simulink model "gm_sampleModel1931_1_sub"  (R2023a)
settings: Solver=VariableStepAuto  StartTime=0.0  StopTime=10.0  RelTol=1e-3
libraries: simulink x3
settings Model: Creator=user1  LastModifiedBy=user1
settings OptimizationCC: BlockReduction=off  ConditionallyExecuteInputs=off
settings DebuggingCC: InheritedTsInSrcMsg=none

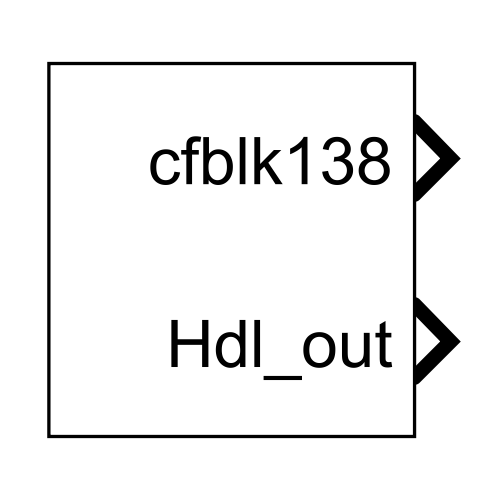
[thumbnail: Simulink's stored preview of the top-level diagram]
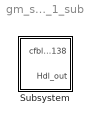
== system gm_sampleModel1931_1_sub ==
  Subsystem : Subsystem

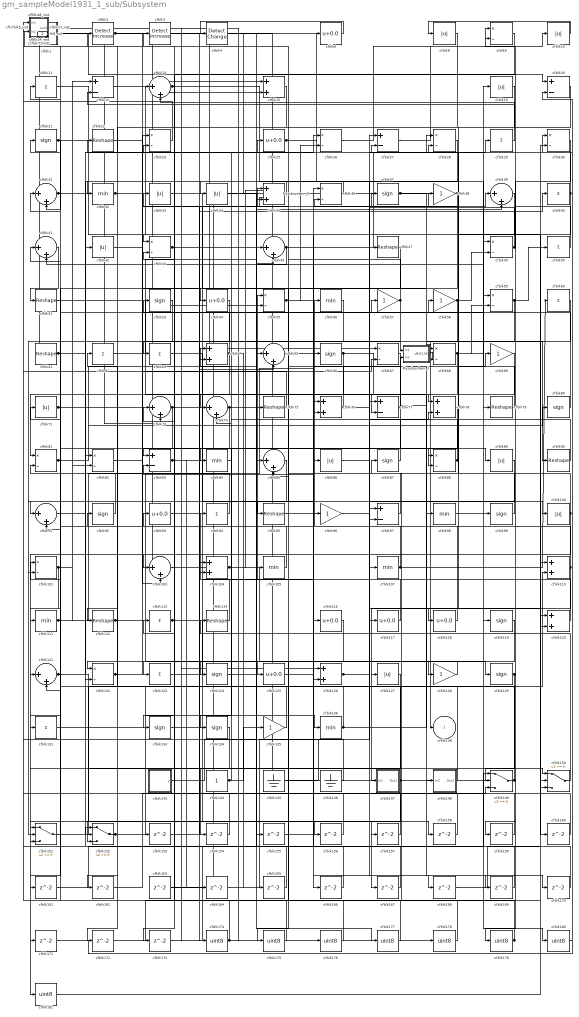
== system gm_sampleModel1931_1_sub/Subsystem ==
  Mysubsystem_1 : Subsystem
  Mysubsystem_5 : Subsystem
  cfblk1 : Subsystem  mask(Compare To Constant){relop=<=, const=double(3), OutDataTypeStr=uint8, ZeroCross=on}
      mask prompts: relop "Simulink:masks:Operator_MP"; const "Simulink:masks:ConstantValue_MP"; OutDataTypeStr "Simulink:masks:OutputDataType_MP"; ZeroCross "Simulink:masks:EnableZerocrossingDetection_MP"
      mask help: Simulink:masks:CompareToConstant_MD
      mask init:
      | OutDataTypeStr = 'uint8';
      | ZeroCross = 'on';
      | blkName = 'sampleModel1931_1_sub/Subsystem/cfblk1';
      | const = double(3);
      | const_str = '3.0';
      | const_val = double(3);
      | relop = '<=';
      | setValue = 'fixdt(0, 8)';
      | str = '<= 3';
      mask TypeOptions relop: == | ~= | < | <= | >= | >
      mask TypeOptions OutDataTypeStr: Simulink:masks:uint8 | Simulink:masks:boolean
      mask Callback ZeroCross: sl('zeroCrossEnable', gcbh);
      mask Display: disp(str)
  cfblk{8,10,19,33..34,42,71,86,89,100,127} (11 alike) : Abs  OutDataTypeStr=uint8  SaturateOnIntegerOverflow=off
  cfblk{9,23,26,28,30,36,43,49,55,59,67..68,81..82,88,101,122} (17 alike) : Product  Inputs=*/  OutDataTypeStr=uint8  RndMeth=Zero  SaturateOnIntegerOverflow=on
  cfblk102_inst : Subsystem
  cfblk{13,31,39,41,45,65,73..74,85,91,103,121} (12 alike) : Sum  Inputs=|++  OutDataTypeStr=uint8
  cfblk{15,35,64,76,78,104,110,120,126} (9 alike) : Sum  OutDataTypeStr=uint8
  cfblk{32,56,84,98,105,107,111,136} (8 alike) : MinMax  OutDataTypeStr=uint8
  cfblk106_inst : Subsystem
  cfblk{11,29,40,50,60,62..63,94,113,123,131} (11 alike) : Sum  Inputs=+  OutDataTypeStr=uint8
  cfblk{22,47,51,61,75,79,90,95,112,114} (10 alike) : Reshape
  cfblk115_inst : Subsystem
  cfblk{6,25,54,93,116..118,125} (8 alike) : Bias  Bias=0.0  SaturateOnIntegerOverflow=off
  cfblk{21,37,53,66,80,87,92,99,119,124,129,133..134} (13 alike) : Signum
  cfblk{12,20,27,77,83,97} (6 alike) : Sum  Inputs=+-  OutDataTypeStr=uint8
  cfblk{38,57..58,69,96,128,135} (7 alike) : Gain  OutDataTypeStr=uint8
  cfblk143 : Subsystem  mask(Counter Free-Running){NumBits=double(16), tsamp=double(-1)}
      mask prompts: NumBits "Simulink:masks:NumberOfBits_MP"; tsamp "Simulink:masks:SampleTime_MP"
      mask help: Simulink:masks:CounterFreeRunning_MD
  cfblk144 : Constant  OutDataTypeStr=uint8  SampleTime=-1
  cfblk145 : Ground
  cfblk146 : Ground
  cfblk147 : Subsystem
  cfblk148 : Subsystem
  cfblk{149..152} (4 alike) : Switch  OutDataTypeStr=uint8  SaturateOnIntegerOverflow=off  InputSameDT=off
  cfblk14_inst : Subsystem
  cfblk{153..173} (21 alike) : Delay  SampleTime=1
  cfblk{174..181} (8 alike) : DataTypeConversion  OutDataTypeStr=uint8  SaturateOnIntegerOverflow=off  RndMeth=Floor
  cfblk17_inst : Subsystem
  cfblk2 : simulink/Logic and Bit Operations/Detect Increase  vinit=0.0  OutDataTypeStr=uint8
      settings: LibrarySourceBlock=|
      | hdlsllib/Logic and Bit
      | Operations/Detect
      | Increase
  cfblk3 : simulink/Logic and Bit Operations/Detect Increase  vinit=0.0  OutDataTypeStr=uint8
      settings: LibrarySourceBlock=|
      | hdlsllib/Logic and Bit
      | Operations/Detect
      | Increase
  cfblk4 : simulink/Logic and Bit Operations/Detect Change  vinit=0  OutDataTypeStr=uint8
      settings: LibrarySourceBlock=|
      | hdlsllib/Logic and Bit
      | Operations/Detect
      | Change
  cfblk48_inst : Subsystem
  cfblk5_inst : Subsystem
  cfblk7_inst : Subsystem
  cfblk138 : Outport  OutDataTypeStr=uint8  SampleTime=1  VectorParamsAs1DForOutWhenUnconnected=off
  Hdl_out : Outport  Port=2  OutDataTypeStr=uint8  SampleTime=1
  wires:
  Mysubsystem_1/1(cfblk138) -> cfblk138/1
  Mysubsystem_5/1(Out1) -> cfblk163/1
  cfblk1/1(y) -> cfblk20/1
  cfblk10/1 -> cfblk8/1
  cfblk100/1 -> cfblk27/2, cfblk181/1
  cfblk101/1 -> cfblk121/1, cfblk82/2
  cfblk102_inst/1(out1) -> cfblk126/1, cfblk67/1
  cfblk103/1 -> cfblk39/1
  cfblk104/1 -> cfblk147/1(In1), Mysubsystem_5/1(In1)
  cfblk105/1 -> cfblk62/1
  cfblk106_inst/1(out1) -> cfblk176/1
  cfblk107/1 -> cfblk56/1, cfblk60/1
  cfblk11/1 -> cfblk43/1
  cfblk110/1 -> cfblk127/1, cfblk81/2
  cfblk111/1 -> cfblk83/2, cfblk12/1
  cfblk112/1 -> cfblk66/1, cfblk125/1
  cfblk113/1 -> cfblk35/1, cfblk150/1
  cfblk114/1 -> cfblk94/1
  cfblk115_inst/1(out1) -> cfblk61/1
  cfblk116/1 -> cfblk175/1
  cfblk117/1 -> cfblk55/1
  cfblk118/1 -> cfblk65/1
  cfblk119/1 -> cfblk123/1
  cfblk12/1 -> cfblk160/1
  cfblk120/1 -> cfblk104/2
  cfblk121/1 -> cfblk42/1, cfblk150/3, cfblk156/1, cfblk11/1
  cfblk122/1 -> cfblk86/1, Mysubsystem_5/2(In2)
  cfblk123/1 -> cfblk36/1
  cfblk124/1 -> cfblk58/1
  cfblk125/1 -> cfblk69/1
  cfblk126/1 -> cfblk78/2, cfblk150/2
  cfblk127/1 -> cfblk154/1
  cfblk128/1 -> cfblk122/1
  cfblk129/1 -> cfblk149/2, cfblk159/1
  cfblk13/1 -> cfblk83/1, cfblk88/2
  cfblk131/1 -> cfblk136/1
  cfblk133/1 -> cfblk167/1
  cfblk134/1 -> cfblk171/1
  cfblk135/1 -> cfblk115_inst/2(in2)
  cfblk136/1 -> cfblk97/1, cfblk5_inst/2(in2), cfblk19/1, cfblk28/2
  cfblk14_inst/1(out1) -> cfblk17_inst/1(in1)
  cfblk143/1(y) -> cfblk45/1
  cfblk144/1 -> cfblk74/2, cfblk135/1
  cfblk145/1 -> cfblk38/1
  cfblk146/1 -> cfblk5_inst/1(in1)
  cfblk147/1(Out1) -> cfblk151/3, cfblk14_inst/1(in1)
  cfblk148/1(Out1) -> cfblk115_inst/1(in1)
  cfblk149/1 -> cfblk92/1, Hdl_out/1
  cfblk15/1 -> cfblk152/3
  cfblk150/1 -> cfblk114/1
  cfblk151/1 -> cfblk85/1
  cfblk152/1 -> cfblk110/2, cfblk153/1
  cfblk153/1 -> cfblk65/2
  cfblk154/1 -> cfblk73/1
  cfblk155/1 -> cfblk76/1
  cfblk156/1 -> cfblk102_inst/1(in1)
  cfblk157/1 -> cfblk121/2
  cfblk158/1 -> cfblk43/2
  cfblk159/1 -> cfblk85/2
  cfblk160/1 -> cfblk104/1
  cfblk161/1 -> cfblk149/1
  cfblk162/1 -> cfblk149/3
  cfblk163/1 -> cfblk126/2
  cfblk164/1 -> cfblk97/2
  cfblk165/1 -> cfblk101/1
  cfblk166/1 -> cfblk152/1
  cfblk167/1 -> cfblk7_inst/2(in2)
  cfblk168/1 -> cfblk120/1
  cfblk169/1 -> cfblk23/2
  cfblk17_inst/1(out1) -> cfblk73/2
  cfblk170/1 -> cfblk14_inst/2(in2)
  cfblk171/1 -> cfblk20/2
  cfblk172/1 -> cfblk110/1
  cfblk173/1 -> cfblk35/2
  cfblk174/1 -> cfblk93/1, cfblk113/1
  cfblk175/1 -> cfblk3/1
  cfblk176/1 -> cfblk41/1
  cfblk177/1 -> cfblk106_inst/1(in1)
  cfblk178/1 -> cfblk106_inst/2(in2)
  cfblk179/1 -> cfblk87/1, cfblk75/1
  cfblk180/1 -> cfblk30/1
  cfblk181/1 -> cfblk30/2
  cfblk19/1 -> cfblk103/1
  cfblk2/1 -> cfblk13/1, cfblk88/1
  cfblk20/1 -> cfblk118/1
  cfblk21/1 -> cfblk31/2, cfblk128/1
  cfblk22/1 -> cfblk54/1
  cfblk23/1 -> cfblk102_inst/2(in2)
  cfblk25/1 -> cfblk117/1, cfblk168/1
  cfblk26/1 -> cfblk10/1
  cfblk27/1 -> cfblk9/1
  cfblk28/1 -> cfblk122/2
  cfblk29/1 -> cfblk13/2
  cfblk3/1 -> cfblk174/1
  cfblk30/1 -> cfblk179/1
  cfblk31/1 -> cfblk103/2, cfblk155/1
  cfblk32/1 -> cfblk112/1, cfblk96/1
  cfblk33/1 -> cfblk68/2
  cfblk34/1 -> cfblk89/1
  cfblk35/1 -> cfblk32/1
  cfblk36/1 -> cfblk34/1
  cfblk37/1 -> cfblk99/1, cfblk90/1
  cfblk38/1 -> cfblk91/1, cfblk36/2, cfblk1/1(u)
  cfblk39/1 -> cfblk77/2
  cfblk4/1 -> cfblk79/1
  cfblk40/1 -> cfblk78/1, cfblk2/1
  cfblk41/1 -> cfblk51/1
  cfblk42/1 -> Mysubsystem_1/1(In1)
  cfblk43/1 -> cfblk45/2, cfblk177/1
  cfblk45/1 -> cfblk41/2, cfblk29/1
  cfblk47/1 -> cfblk95/1
  cfblk48_inst/1(out1) -> cfblk178/1, cfblk55/2
  cfblk49/1 -> cfblk27/1, cfblk9/2
  cfblk5_inst/1(out1) -> cfblk15/1, cfblk105/1
  cfblk50/1 -> cfblk12/2
  cfblk51/1 -> cfblk148/1(In1)
  cfblk53/1 -> cfblk111/1
  cfblk54/1 -> cfblk151/1
  cfblk55/1 -> cfblk47/1, cfblk26/2
  cfblk56/1 -> cfblk173/1
  cfblk57/1 -> cfblk48_inst/2(in2), cfblk107/1
  cfblk58/1 -> cfblk151/2, cfblk49/2
  cfblk59/1 -> cfblk162/1, cfblk161/1, cfblk50/1
  cfblk6/1 -> cfblk4/1
  cfblk60/1 -> cfblk68/1
  cfblk61/1 -> cfblk158/1, cfblk157/1
  cfblk62/1 -> cfblk6/1
  cfblk63/1 -> cfblk166/1
  cfblk64/1 -> cfblk74/1, cfblk53/1, cfblk165/1
  cfblk65/1 -> cfblk116/1
  cfblk66/1 -> cfblk81/1, cfblk98/1
  cfblk67/1 -> cfblk170/1
  cfblk68/1 -> cfblk119/1, cfblk59/2, cfblk172/1
  cfblk69/1 -> cfblk76/2
  cfblk7_inst/1(out1) -> cfblk15/2
  cfblk71/1 -> cfblk25/1, cfblk67/2
  cfblk73/1 -> cfblk37/1, cfblk152/2
  cfblk74/1 -> cfblk91/2, cfblk49/1
  cfblk75/1 -> cfblk48_inst/1(in1)
  cfblk76/1 -> cfblk17_inst/2(in2), cfblk120/2
  cfblk77/1 -> cfblk33/1, cfblk124/1
  cfblk78/1 -> cfblk131/1
  cfblk79/1 -> cfblk57/1
  cfblk8/1 -> cfblk133/1
  cfblk80/1 -> cfblk21/1
  cfblk81/1 -> cfblk80/1, cfblk39/2, cfblk31/1
  cfblk82/1 -> cfblk59/1
  cfblk83/1 -> cfblk28/1, cfblk164/1, Mysubsystem_1/2(In2)
  cfblk84/1 -> cfblk64/1
  cfblk85/1 -> cfblk101/2
  cfblk86/1 -> cfblk129/1
  cfblk87/1 -> cfblk77/1
  cfblk88/1 -> cfblk64/2, cfblk84/1
  cfblk89/1 -> cfblk134/1
  cfblk9/1 -> cfblk63/1
  cfblk90/1 -> cfblk23/1
  cfblk91/1 -> cfblk26/1
  cfblk92/1 -> cfblk82/1
  cfblk93/1 -> cfblk40/1
  cfblk94/1 -> cfblk71/1
  cfblk95/1 -> cfblk169/1
  cfblk96/1 -> cfblk100/1
  cfblk97/1 -> cfblk7_inst/1(in1)
  cfblk98/1 -> cfblk180/1
  cfblk99/1 -> cfblk22/1

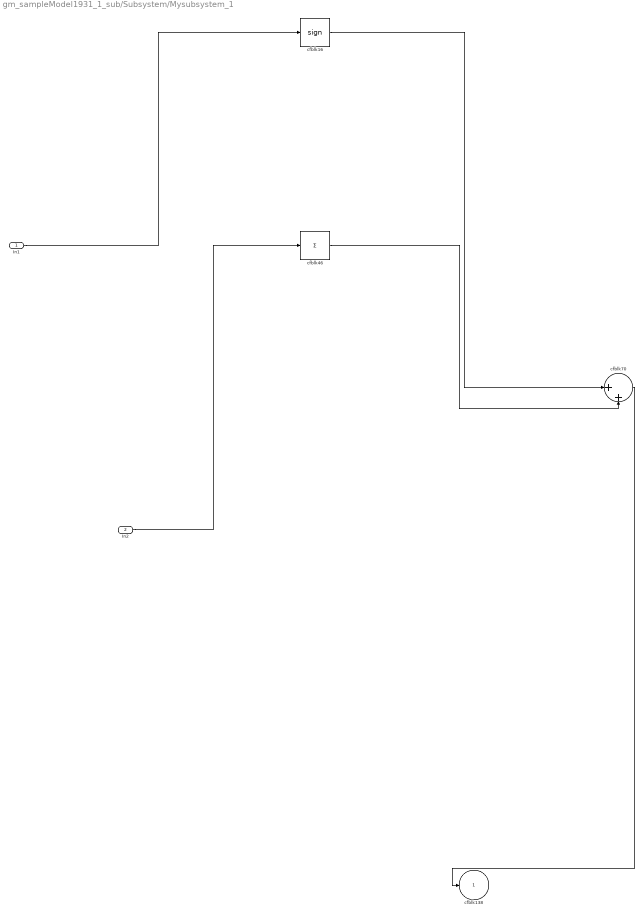
== system gm_sampleModel1931_1_sub/Subsystem/Mysubsystem_1 ==
  In1 : Inport  OutDataTypeStr=uint8  PortDimensions=1  SampleTime=1
  In2 : Inport  Port=2  OutDataTypeStr=uint8  PortDimensions=1  SampleTime=1
  cfblk16 : Signum
  cfblk46 : Sum  Inputs=+
  cfblk70 : Sum  Inputs=|++
  cfblk138 : Outport  SampleTime=1  VectorParamsAs1DForOutWhenUnconnected=off
  wires:
  In1/1 -> cfblk16/1
  In2/1 -> cfblk46/1
  cfblk16/1 -> cfblk70/1
  cfblk46/1 -> cfblk70/2
  cfblk70/1 -> cfblk138/1

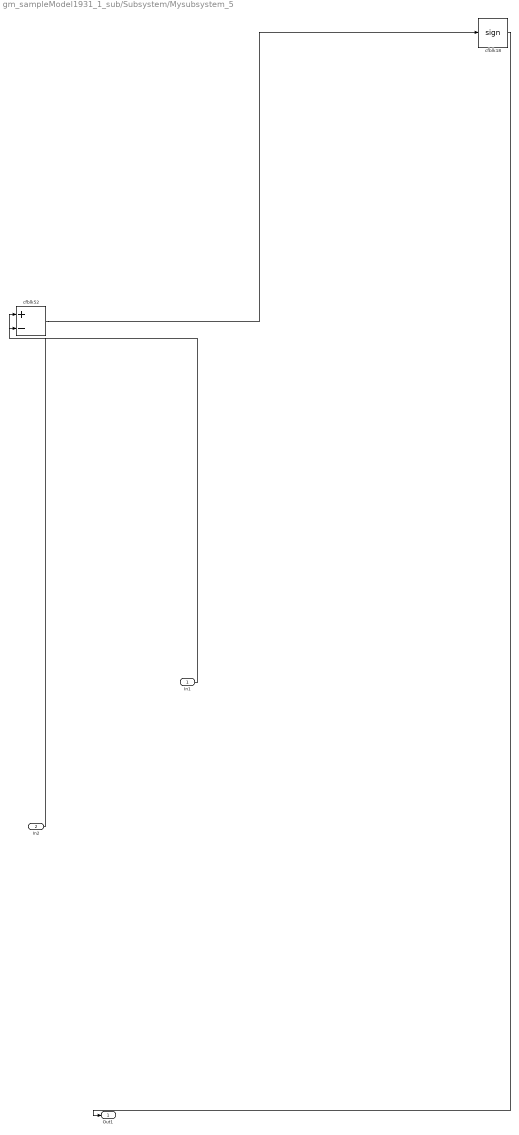
== system gm_sampleModel1931_1_sub/Subsystem/Mysubsystem_5 ==
  In1 : Inport  OutDataTypeStr=uint8  PortDimensions=1  SampleTime=1
  In2 : Inport  Port=2  OutDataTypeStr=uint8  PortDimensions=1  SampleTime=1
  cfblk18 : Signum
  cfblk52 : Sum  Inputs=+-
  Out1 : Outport  SampleTime=1
  wires:
  In1/1 -> cfblk52/1
  In2/1 -> cfblk52/2
  cfblk18/1 -> Out1/1
  cfblk52/1 -> cfblk18/1

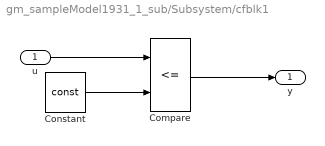
== system gm_sampleModel1931_1_sub/Subsystem/cfblk1 ==
  u : Inport  OutDataTypeStr=uint8  SampleTime=1
  Compare : RelationalOperator  Operator=<=  OutDataTypeStr=fixdt(0, 8)
  Constant : Constant  DisableCoverage=on  Value=const  OutDataTypeStr=Inherit: Inherit via back propagation  SampleTime=-1
  y : Outport  SampleTime=1
  wires:
  u/1 -> Compare/1
  Compare/1 -> y/1
  Constant/1 -> Compare/2

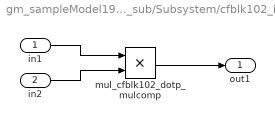
== system gm_sampleModel1931_1_sub/Subsystem/cfblk102_inst ==
  in1 : Inport  OutDataTypeStr=uint8  SampleTime=1
  in2 : Inport  Port=2  OutDataTypeStr=uint8  SampleTime=1
  mul_cfblk102_dotp_mulcomp : Product  Inputs=**  OutDataTypeStr=uint8  SampleTime=1
  out1 : Outport  OutDataTypeStr=uint8  SampleTime=1
  wires:
  in1/1 -> mul_cfblk102_dotp_mulcomp/1
  in2/1 -> mul_cfblk102_dotp_mulcomp/2
  mul_cfblk102_dotp_mulcomp/1 -> out1/1

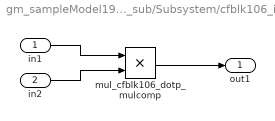
== system gm_sampleModel1931_1_sub/Subsystem/cfblk106_inst ==
  in1 : Inport  OutDataTypeStr=uint8  SampleTime=1
  in2 : Inport  Port=2  OutDataTypeStr=uint8  SampleTime=1
  mul_cfblk106_dotp_mulcomp : Product  Inputs=**  OutDataTypeStr=uint8  SampleTime=1
  out1 : Outport  OutDataTypeStr=uint8  SampleTime=1
  wires:
  in1/1 -> mul_cfblk106_dotp_mulcomp/1
  in2/1 -> mul_cfblk106_dotp_mulcomp/2
  mul_cfblk106_dotp_mulcomp/1 -> out1/1

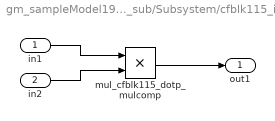
== system gm_sampleModel1931_1_sub/Subsystem/cfblk115_inst ==
  in1 : Inport  OutDataTypeStr=uint8  SampleTime=1
  in2 : Inport  Port=2  OutDataTypeStr=uint8  SampleTime=1
  mul_cfblk115_dotp_mulcomp : Product  Inputs=**  OutDataTypeStr=uint8  SampleTime=1
  out1 : Outport  OutDataTypeStr=uint8  SampleTime=1
  wires:
  in1/1 -> mul_cfblk115_dotp_mulcomp/1
  in2/1 -> mul_cfblk115_dotp_mulcomp/2
  mul_cfblk115_dotp_mulcomp/1 -> out1/1

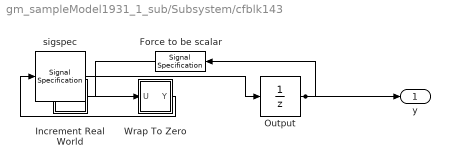
== system gm_sampleModel1931_1_sub/Subsystem/cfblk143 ==
  Force to be scalar : SignalSpecification  DisableCoverage=on  Dimensions=1
  Increment Real World : Subsystem  mask(Real World Value Increment){}
      mask help: Simulink:masks:RealWorldValueIncrement_MD
      mask Display: disp('V++')
  Output : UnitDelay  InitialCondition=0.0  SampleTime=tsamp  HasFrameUpgradeWarning=on
  Wrap To Zero : Subsystem  mask(Wrap To Zero){Threshold=double(65535)}
      mask prompts: Threshold "Simulink:masks:Threshold_MP"
      mask help: Simulink:masks:WrapToZero_MD
  sigspec : SignalSpecification  OutDataTypeStr=uint16  Dimensions=1
  y : Outport  SampleTime=1
  wires:
  Force to be scalar/1 -> Increment Real World/1(u)
  Increment Real World/1(y) -> Wrap To Zero/1(U)
  Output/1 -> Force to be scalar/1, y/1
  Wrap To Zero/1(Y) -> sigspec/1
  sigspec/1 -> Output/1

== system gm_sampleModel1931_1_sub/Subsystem/cfblk147 ==
  In1 : Inport  OutDataTypeStr=uint8  PortDimensions=1  SampleTime=1
  Out1 : Outport  SampleTime=1
  wires:
  In1/1 -> Out1/1

== system gm_sampleModel1931_1_sub/Subsystem/cfblk148 ==
  In1 : Inport  OutDataTypeStr=uint8  PortDimensions=1  SampleTime=1
  Out1 : Outport  SampleTime=1
  wires:
  In1/1 -> Out1/1

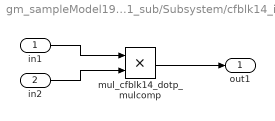
== system gm_sampleModel1931_1_sub/Subsystem/cfblk14_inst ==
  in1 : Inport  OutDataTypeStr=uint8  SampleTime=1
  in2 : Inport  Port=2  OutDataTypeStr=uint8  SampleTime=1
  mul_cfblk14_dotp_mulcomp : Product  Inputs=**  OutDataTypeStr=uint8  SampleTime=1
  out1 : Outport  OutDataTypeStr=uint8  SampleTime=1
  wires:
  in1/1 -> mul_cfblk14_dotp_mulcomp/1
  in2/1 -> mul_cfblk14_dotp_mulcomp/2
  mul_cfblk14_dotp_mulcomp/1 -> out1/1

== system gm_sampleModel1931_1_sub/Subsystem/cfblk17_inst ==
  in1 : Inport  OutDataTypeStr=uint8  SampleTime=1
  in2 : Inport  Port=2  OutDataTypeStr=uint8  SampleTime=1
  mul_cfblk17_dotp_mulcomp : Product  Inputs=**  OutDataTypeStr=uint8  SampleTime=1
  out1 : Outport  OutDataTypeStr=uint8  SampleTime=1
  wires:
  in1/1 -> mul_cfblk17_dotp_mulcomp/1
  in2/1 -> mul_cfblk17_dotp_mulcomp/2
  mul_cfblk17_dotp_mulcomp/1 -> out1/1

== system gm_sampleModel1931_1_sub/Subsystem/cfblk48_inst ==
  in1 : Inport  OutDataTypeStr=uint8  SampleTime=1
  in2 : Inport  Port=2  OutDataTypeStr=uint8  SampleTime=1
  mul_cfblk48_dotp_mulcomp : Product  Inputs=**  OutDataTypeStr=uint8  SampleTime=1
  out1 : Outport  OutDataTypeStr=uint8  SampleTime=1
  wires:
  in1/1 -> mul_cfblk48_dotp_mulcomp/1
  in2/1 -> mul_cfblk48_dotp_mulcomp/2
  mul_cfblk48_dotp_mulcomp/1 -> out1/1

== system gm_sampleModel1931_1_sub/Subsystem/cfblk5_inst ==
  in1 : Inport  OutDataTypeStr=uint8  SampleTime=1
  in2 : Inport  Port=2  OutDataTypeStr=uint8  SampleTime=1
  mul_cfblk5_dotp_mulcomp : Product  Inputs=**  OutDataTypeStr=uint8  SampleTime=1
  out1 : Outport  OutDataTypeStr=uint8  SampleTime=1
  wires:
  in1/1 -> mul_cfblk5_dotp_mulcomp/1
  in2/1 -> mul_cfblk5_dotp_mulcomp/2
  mul_cfblk5_dotp_mulcomp/1 -> out1/1

== system gm_sampleModel1931_1_sub/Subsystem/cfblk7_inst ==
  in1 : Inport  OutDataTypeStr=uint8  SampleTime=1
  in2 : Inport  Port=2  OutDataTypeStr=uint8  SampleTime=1
  mul_cfblk7_dotp_mulcomp : Product  Inputs=**  OutDataTypeStr=uint8  SampleTime=1
  out1 : Outport  OutDataTypeStr=uint8  SampleTime=1
  wires:
  in1/1 -> mul_cfblk7_dotp_mulcomp/1
  in2/1 -> mul_cfblk7_dotp_mulcomp/2
  mul_cfblk7_dotp_mulcomp/1 -> out1/1

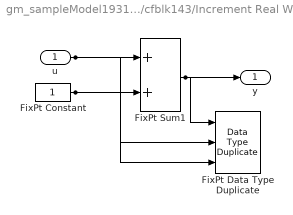
== system gm_sampleModel1931_1_sub/Subsystem/cfblk143/Increment Real World ==
  u : Inport  OutDataTypeStr=uint16  SampleTime=1
  FixPt Constant : Constant  DisableCoverage=on  OutDataTypeStr=Inherit: Inherit via back propagation  SampleTime=-1
  FixPt Data Type Duplicate : DataTypeDuplicate  DisableCoverage=on  NumInputPorts=3
  FixPt Sum1 : Sum  InputSameDT=on  OutDataTypeStr=Inherit: Inherit via back propagation  LockScale=on
  y : Outport  SampleTime=1
  wires:
  u/1 -> FixPt Sum1/1, FixPt Data Type Duplicate/2
  FixPt Constant/1 -> FixPt Sum1/2, FixPt Data Type Duplicate/3
  FixPt Sum1/1 -> FixPt Data Type Duplicate/1, y/1

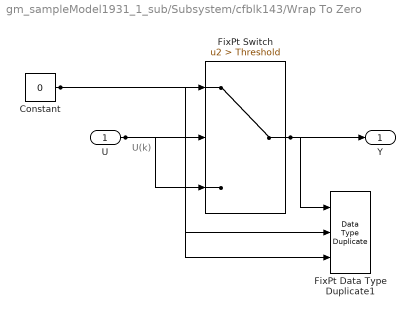
== system gm_sampleModel1931_1_sub/Subsystem/cfblk143/Wrap To Zero ==
  note: U(k)
  U : Inport  OutDataTypeStr=uint16  SampleTime=1
  Constant : Constant  DisableCoverage=on  Value=0  OutDataTypeStr=Inherit: Inherit via back propagation  SampleTime=-1
  FixPt Data Type Duplicate1 : DataTypeDuplicate  DisableCoverage=on  NumInputPorts=3
  FixPt Switch : Switch  Criteria=u2 > Threshold  Threshold=Threshold  OutDataTypeStr=Inherit: Inherit via back propagation  ZeroCross=off  SaturateOnIntegerOverflow=off  InputSameDT=off
  Y : Outport  SampleTime=1
  wires:
  U/1 -> FixPt Switch/3, FixPt Switch/2, FixPt Data Type Duplicate1/2
  Constant/1 -> FixPt Switch/1, FixPt Data Type Duplicate1/3
  FixPt Switch/1 -> FixPt Data Type Duplicate1/1, Y/1
